simulink model "is95revchdetection"  (Simulink 4.00)
settings: Solver=VariableStepDiscrete  SolverMode=SingleTasking  StartTime=0.0  StopTime=2  RelTol=1e-3  AbsTol=1e-6
undefined symbols (not defined in the file or in its folder): slcm
libraries: cdmalib x3, dspbdsp2 x3, dspsrcs2 x2, commchan x2, commsink x1
settings Model: Creator=rkumar  LastModifiedBy=akansal  SaveTime=off  SaveOutput=off  LimitDataPoints=off  ExtModeTrigMode=oneshot  ExtModeArmWhenConnect=off  BlockReductionOpt=off

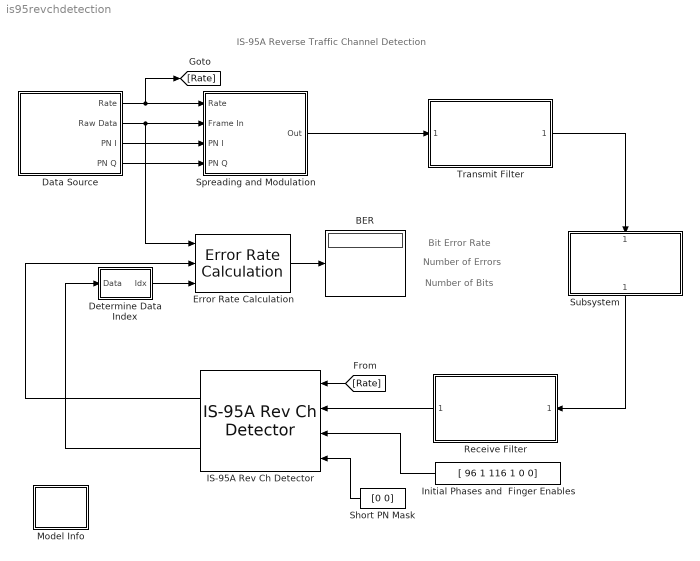
== system is95revchdetection ==
  note: IS-95A Reverse Traffic Channel Detection
  note: Bit Error Rate
  note: Number of Errors
  note: Number of Bits
  " Spreading and Modulation " : Subsystem
      settings: RTWFcnNameOpts=Auto  RTWFileNameOpts=Auto
  BER : Display
      settings: Format=short
  Data Source : Subsystem
      settings: RTWFcnNameOpts=Auto  RTWFileNameOpts=Auto
  Determine Data Index : Subsystem
      settings: RTWFcnNameOpts=Auto  RTWFileNameOpts=Auto
  Error Rate Calculation : commsink/Error Rate Calculation  N=2*576  st_delay=2*576  cp_mode=Select samples from port  subframe=[]  PMode=Port  WsName=ErrorVec  RsMode2=off
  IS-95A Rev Ch Detector : cdmalib/IS-95A Base Station Receiver/IS-95A Rev Ch Detector  Orientation=left  chType=Traffic  wlshOrd=6  lngcd_mask=1  overSamplRate=8  sampTime=1/(50*384)
  Initial Phases and  Finger Enables : Constant  Orientation=left  Value=[ 96 1 116 1 0 0]
  Model Info : Subsystem  LoadFcn=slcm LoadBlock;  InitFcn=slcm('UpdateAllCMBlocksInThisModelInit')  mask(CMBlock){InitialSaveTempField=, InitialBlockCM=none, BlockCM=none, Frame=on, SaveTempField=, DisplayStringWithTags=Info, MaskDisplayString=Info, HorizontalTextAlignment=Center, LeftAlignmentValue=0.5, SourceBlockDiagram=is95revchdetection, TagMaxNumber=20, CMTag1=, CMTag2=, CMTag3=, CMTag4=, CMTag5=, CMTag6=, CMTag7=, CMTag8=, CMTag9=, CMTag10=, CMTag11=, CMTag12=, CMTag13=, CMTag14=, CMTag15=, CMTag16=, CMTag17=, CMTag18=, CMTag19=, CMTag20=}
      mask help: This block allows revision control information to be displayed within the model.
      settings: CopyFcn=slcm CopyBlock;  DeleteFcn=slcm Cancel;  PostSaveFcn=slcm('UpdateAllCMBlocksInThisModel')  NameChangeFcn=slcm Rename;  OpenFcn=cdmademohelp;  RTWFcnNameOpts=Auto  RTWFileNameOpts=Auto
      mask Display: text(str2num(LeftAlignmentValue), 0.5, MaskDisplayString, 'HorizontalAlignment', HorizontalTextAlignment)
  Receive Filter : Subsystem  Orientation=left  mask(FIR Pulse Shaping Filter){N=1}
      mask prompts: N "Interpolation factor:"
      mask help: The length of the FIR filter is the duration of 12 PN sequence chips. The coefficient spacing and the sample time of this filter is one-eighth of the PN sequence chip duration, resulting in a total of 96 coefficients. The filter introduces a delay of 48 samples.
      mask init:
      | load txfiltx8.mat;
      | h = (TxFiltCoefx8*N)/8;
      settings: RTWFcnNameOpts=Auto  RTWFileNameOpts=Auto
      mask Display: plot( 1:prod( size( h)), h);
  Short PN Mask : Constant  Orientation=left  Value=[0 0]
  Subsystem : Subsystem  Orientation=down
      settings: RTWFcnNameOpts=Auto  RTWFileNameOpts=Auto
      mask Display: disp('Rayleigh Multipath\n and  AWGN\nChannel')
  Transmit Filter : Subsystem  mask(FIR Pulse Shaping Filter){N=1}
      mask prompts: N "Interpolation factor:"
      mask help: The length of the FIR filter is the duration of 12 PN sequence chips. The coefficient spacing and the sample time of this filter is one-eighth of the PN sequence chip duration, resulting in a total of 96 coefficients. The filter introduces a delay of 48 samples.
      mask init:
      | load txfiltx8.mat;
      | h = (TxFiltCoefx8*N);
      settings: RTWFcnNameOpts=Auto  RTWFileNameOpts=Auto
      mask Display: plot( 1:prod( size( h)), h);
  wires:
  " Spreading and Modulation "/1("Out ") -> Transmit Filter/1("   ")
  Transmit Filter/1(" ") -> Subsystem/1(" ")
  Data Source/3(PN I) -> " Spreading and Modulation "/3(PN I)
  Data Source/4(PN Q) -> " Spreading and Modulation "/4(PN Q)
  Data Source/1(Rate) -> " Spreading and Modulation "/1(Rate), [Rate]
  Subsystem/1("  ") -> Receive Filter/1("   ")
  Short PN Mask/1 -> IS-95A Rev Ch Detector/4
  [Rate] -> IS-95A Rev Ch Detector/1
  Receive Filter/1(" ") -> IS-95A Rev Ch Detector/2
  Initial Phases and  Finger Enables/1 -> IS-95A Rev Ch Detector/3
  Determine Data Index/1(Idx) -> Error Rate Calculation/3
  Error Rate Calculation/1 -> BER/1
  IS-95A Rev Ch Detector/2 -> Determine Data Index/1(Data)
  IS-95A Rev Ch Detector/1 -> Error Rate Calculation/2
  Data Source/2(Raw Data) -> " Spreading and Modulation "/2(Frame In), Error Rate Calculation/1

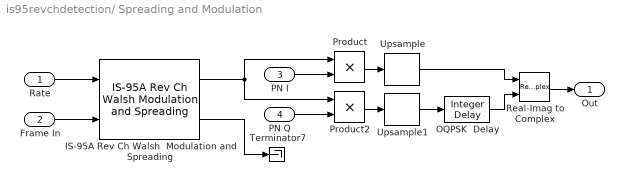
== system is95revchdetection/ Spreading and Modulation  ==
  Rate : Inport  Port=1
  Frame In : Inport  Port=2
  PN I : Inport  Port=3
  PN Q : Inport  Port=4
  IS-95A Rev Ch Walsh  Modulation and Spreading : cdmalib/IS-95A Mobile Station Transmitter/IS-95A Rev Ch Walsh Modulation and Spreading  chType=Traffic  lngCdMask=1  wlshOrd=6  sampTime=1/(50*384)
  OQPSK  Delay : dspbdsp2/Integer Delay  delay=4  ic=0  frame=on  df=on  numChans=1
  Product : Product  Inputs=2  Multiplication=Element-wise(.*)  SaturateOnIntegerOverflow=on
  Product2 : Product  Inputs=2  Multiplication=Element-wise(.*)  SaturateOnIntegerOverflow=on
  Real-Imag to Complex : RealImagToComplex  Input=RealAndImag  ConstantPart=0
  Terminator7 : Terminator
  Upsample : dspbdsp2/Upsample  N=8  phase=0  ic=0  frame=on  nchans=1  mode=Maintain input frame rate
  Upsample1 : dspbdsp2/Upsample  N=8  phase=0  ic=0  frame=on  nchans=1  mode=Maintain input frame rate
  "Out " : Outport  Port=1
  wires:
  IS-95A Rev Ch Walsh  Modulation and Spreading/1 -> Product/1, Product2/1
  Rate/1 -> IS-95A Rev Ch Walsh  Modulation and Spreading/1
  PN I/1 -> Product/2
  Frame In/1 -> IS-95A Rev Ch Walsh  Modulation and Spreading/2
  PN Q/1 -> Product2/2
  Product/1 -> Upsample/1
  Product2/1 -> Upsample1/1
  Upsample1/1 -> OQPSK  Delay/1
  OQPSK  Delay/1 -> Real-Imag to Complex/2
  Upsample/1 -> Real-Imag to Complex/1
  Real-Imag to Complex/1 -> "Out "/1
  IS-95A Rev Ch Walsh  Modulation and Spreading/2 -> Terminator7/1

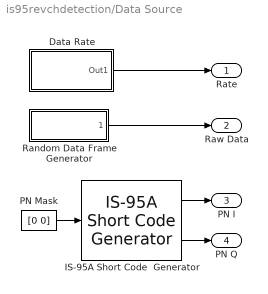
== system is95revchdetection/Data Source ==
  Data Rate : Subsystem  mask{rate=Full}
      mask prompts: rate "Data Rate"
      settings: RTWFcnNameOpts=Auto  RTWFileNameOpts=Auto
      mask StyleString: popup(Full|Half|Quarter|One-Eighth)
      mask Display: disp('Mobile Station \n Transmitter \nData Rate')
  IS-95A Short Code  Generator : cdmalib/IS-95A Common/IS-95A Short Code Generator  numOut=64  sampTime=1/(50*384)
  PN Mask : Constant  Value=[0 0]
  Random Data Frame Generator : Subsystem  mask(Random Binary Frame Generator){seed=119940, Ts=1/(50*576), N=576}
      mask prompts: seed "Initial seed:"; Ts "Sample time (sec):"; N "Output frame size:"
      mask help:
      | Generate a random frame of binary integers. The output frame period is
      | (Sample time) * (Output frame size).
      settings: RTWFcnNameOpts=Auto  RTWFileNameOpts=Auto
      mask Display: plot(0,0,100,100,[95,90,90,80,80,60,60,30,30,20,20,10,10,5],[25,25,75,75,25,25,75,75,25,25,75,75,25,25]);
  Rate : Outport  Port=1  InitialOutput=0
  Raw Data : Outport  Port=2  InitialOutput=0
  PN I : Outport  Port=3  InitialOutput=0
  PN Q : Outport  Port=4  InitialOutput=0
  wires:
  Data Rate/1(Out1) -> Rate/1
  PN Mask/1 -> IS-95A Short Code  Generator/1
  IS-95A Short Code  Generator/1 -> PN I/1
  IS-95A Short Code  Generator/2 -> PN Q/1
  Random Data Frame Generator/1(" ") -> Raw Data/1

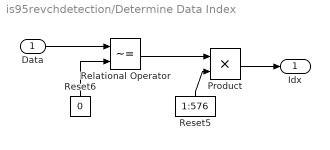
== system is95revchdetection/Determine Data Index ==
  Data : Inport  Port=1
  Product : Product  Inputs=2  Multiplication=Element-wise(.*)  SaturateOnIntegerOverflow=on
  Relational Operator : RelationalOperator  Operator=~=
  Reset5 : Constant  Orientation=up  Value=1:576
  Reset6 : Constant  Orientation=up  Value=0
  Idx : Outport  Port=1
  wires:
  Reset6/1 -> Relational Operator/2
  Relational Operator/1 -> Product/1
  Reset5/1 -> Product/2
  Data/1 -> Relational Operator/1
  Product/1 -> Idx/1

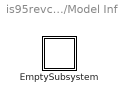
== system is95revchdetection/Model Info ==
  EmptySubsystem : Subsystem
      settings: RTWFcnNameOpts=Auto  RTWFileNameOpts=Auto

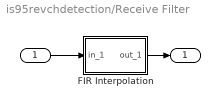
== system is95revchdetection/Receive Filter ==
  "   " : Inport  Port=1
  FIR Interpolation : Subsystem  mask(FIR Interpolation){h=h, L=N, frame=on, numChans=1, framing=Maintain input frame rate}
      mask prompts: h "FIR filter coefficients:"; L "Interpolation factor:"; frame "Frame-based inputs"; numChans "Number of channels:"
      mask help: Upsample input signal by an integer factor, then apply an FIR filter. Implemented using an efficient polyphase interpolation structure. The filter coefficients are scaled by the interpolation factor.
      mask init:
      | outputBufInitCond = 0;
      | [str,numChans] = dspblkupfir('setup1',numChans);
      | [h,framing,str]= dspblkupfir('setup2',h,L,framing);
      settings: RTWFcnNameOpts=Auto  RTWFileNameOpts=Auto
      mask Help: web(dspbhelp);
      mask StyleString: edit,edit,checkbox,edit,popup(Maintain input frame size|Maintain input frame rate)
      mask CallbackString: ||dspblkupfir||
      mask Display: disp(str)
  " " : Outport  Port=1
  wires:
  "   "/1 -> FIR Interpolation/1(in_1)
  FIR Interpolation/1(out_1) -> " "/1

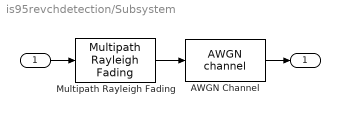
== system is95revchdetection/Subsystem ==
  " " : Inport  Port=1
  AWGN Channel : commchan/AWGN channel  seed=123456  noiseMode="Signal to noise ratio  (Es/No)"  EsNodB=10  SNRdB=10  Ps=1  Tsym=1/1228800  variance=1  FrameBased=on  nChans=1
  Multipath Rayleigh Fading : commchan/Multipath Rayleigh Fading  Fd=14.07  simTs=1/(1228800*8)  delayVec=[0 2e-6]  gainVecdB=[0 0]  normGain=on  Seed=831029
  "  " : Outport  Port=1
  wires:
  Multipath Rayleigh Fading/1 -> AWGN Channel/1
  " "/1 -> Multipath Rayleigh Fading/1
  AWGN Channel/1 -> "  "/1

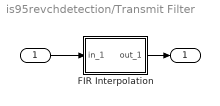
== system is95revchdetection/Transmit Filter ==
  "   " : Inport  Port=1
  FIR Interpolation : Subsystem  mask(FIR Interpolation){h=h, L=N, frame=on, numChans=1, framing=Maintain input frame rate}
      mask prompts: h "FIR filter coefficients:"; L "Interpolation factor:"; frame "Frame-based inputs"; numChans "Number of channels:"
      mask help: Upsample input signal by an integer factor, then apply an FIR filter. Implemented using an efficient polyphase interpolation structure. The filter coefficients are scaled by the interpolation factor.
      mask init:
      | outputBufInitCond = 0;
      | [str,numChans] = dspblkupfir('setup1',numChans);
      | [h,framing,str]= dspblkupfir('setup2',h,L,framing);
      settings: RTWFcnNameOpts=Auto  RTWFileNameOpts=Auto
      mask Help: web(dspbhelp);
      mask StyleString: edit,edit,checkbox,edit,popup(Maintain input frame size|Maintain input frame rate)
      mask CallbackString: ||dspblkupfir||
      mask Display: disp(str)
  " " : Outport  Port=1
  wires:
  FIR Interpolation/1(out_1) -> " "/1
  "   "/1 -> FIR Interpolation/1(in_1)

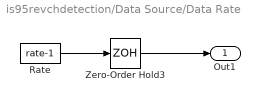
== system is95revchdetection/Data Source/Data Rate ==
  Rate : Constant  Value=rate-1
  Zero-Order Hold3 : ZeroOrderHold  SampleTime=1/50
  Out1 : Outport  Port=1  InitialOutput=0
  wires:
  Zero-Order Hold3/1 -> Out1/1
  Rate/1 -> Zero-Order Hold3/1

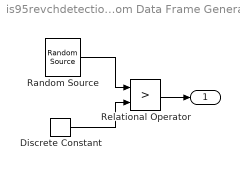
== system is95revchdetection/Data Source/Random Data Frame Generator ==
  Discrete Constant : dspsrcs2/Discrete Constant  Value=0.5  Ts=Ts*N
  Random Source : dspsrcs2/Random Source  SrcType=Uniform  Min=0  Max=1  Mean=0  Var=1  Seed=seed  SampMode=Discrete  Inherit=off  SampTime=Ts  SampFrame=N  OutComplex=Real
  Relational Operator : RelationalOperator  Operator=>
  " " : Outport  Port=1
  wires:
  Random Source/1 -> Relational Operator/1
  Discrete Constant/1 -> Relational Operator/2
  Relational Operator/1 -> " "/1

== system is95revchdetection/Model Info/EmptySubsystem ==

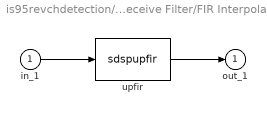
== system is95revchdetection/Receive Filter/FIR Interpolation ==
  in_1 : Inport  Port=1
  upfir : S-Function  FunctionName=sdspupfir  Parameters=h,L,numChans,framing,outputBufInitCond  PortCounts=[]  SFunctionModules=''
  out_1 : Outport  Port=1  InitialOutput=0
  wires:
  upfir/1 -> out_1/1
  in_1/1 -> upfir/1

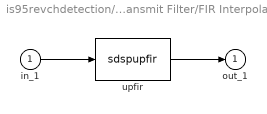
== system is95revchdetection/Transmit Filter/FIR Interpolation ==
  in_1 : Inport  Port=1
  upfir : S-Function  FunctionName=sdspupfir  Parameters=h,L,numChans,framing,outputBufInitCond  PortCounts=[]  SFunctionModules=''
  out_1 : Outport  Port=1  InitialOutput=0
  wires:
  in_1/1 -> upfir/1
  upfir/1 -> out_1/1
